simulink model "MKZ_Model"  (R2020a)
settings: Solver=FixedStepAuto  StartTime=0.0  StopTime=RunTime  FixedStep=SampleTime  RelTol=1e-3
PreLoadFcn:
  | load('BrkEngMaps.mat');
values from neighbouring files (symbols this model uses):
  InitVel = VehSpeed.Data(1)    [TestCarModel.m]
  SampleTime = 0.05    [TestCarModel.m]
undefined symbols (not defined in the file or in its folder): BrakeZ, DiscIntNeverNeededParam, EngineZ, XbrkPts, XengPts, YbrkPts, YengPts
libraries: dspstat3 x1
settings Model: Creator=VVK Desktop1  LastModifiedBy=VVK

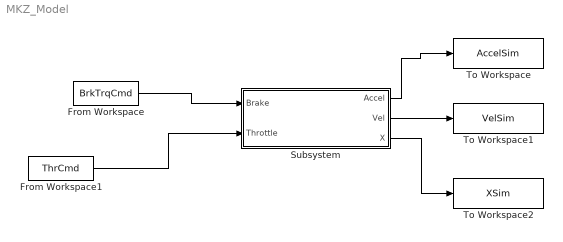
== system MKZ_Model ==
  From Workspace : FromWorkspace  VariableName=BrkTrqCmd  SampleTime=SampleTime
  From Workspace1 : FromWorkspace  VariableName=ThrCmd  SampleTime=SampleTime
  Subsystem : Subsystem
  To Workspace : ToWorkspace  VariableName=AccelSim  SaveFormat=Timeseries  SampleTime=-1
  To Workspace1 : ToWorkspace  VariableName=VelSim  SaveFormat=Timeseries  SampleTime=-1
  To Workspace2 : ToWorkspace  VariableName=XSim  SaveFormat=Timeseries  SampleTime=-1
  wires:
  From Workspace/1 -> Subsystem/1(Brake)
  From Workspace1/1 -> Subsystem/2(Throttle)
  Subsystem/2(Vel) -> To Workspace1/1
  Subsystem/3(X) -> To Workspace2/1
  Subsystem/1(Accel) -> To Workspace/1

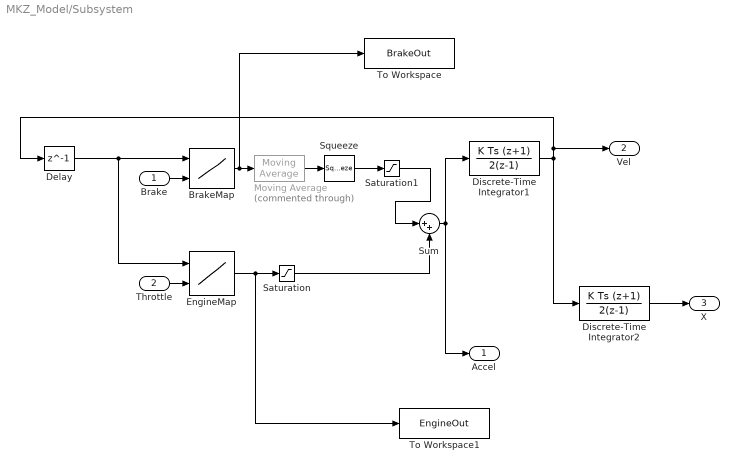
== system MKZ_Model/Subsystem ==
  Brake : Inport
  Throttle : Inport  Port=2
  BrakeMap : Lookup_n-D  BreakpointsForDimension1=XbrkPts  BreakpointsForDimension2=YbrkPts  Table=BrakeZ  InternalRulePriority=Speed  RndMeth=Simplest  InputSameDT=on
  Delay : Delay  DelayLength=1  InitialCondition=InitVel
  Discrete-Time Integrator1 : DiscreteIntegrator  IntegratorMethod=Integration: Trapezoidal  InitialCondition=InitVel  SampleTime=-1  LimitOutput=on  LowerSaturationLimit=0  ICPrevOutput=DiscIntNeverNeededParam  ICPrevScaledInput=DiscIntNeverNeededParam
  Discrete-Time Integrator2 : DiscreteIntegrator  IntegratorMethod=Integration: Trapezoidal  SampleTime=-1  LimitOutput=on  LowerSaturationLimit=0  ICPrevOutput=DiscIntNeverNeededParam  ICPrevScaledInput=DiscIntNeverNeededParam
  EngineMap : Lookup_n-D  BreakpointsForDimension1=XengPts  BreakpointsForDimension2=YengPts  Table=EngineZ  InternalRulePriority=Speed  RndMeth=Simplest  InputSameDT=on
  Moving Average : dspstat3/Moving Average  Commented=through  Method=Sliding window  ForgettingFactorPort=off  SpecifyWindowLength=on  WindowLength=4  ForgettingFactor=0.9  SimulateUsing=Code generation
  Saturation : Saturate  UpperLimit=3.5  LowerLimit=-0.25
  Saturation1 : Saturate  UpperLimit=0  LowerLimit=-3.5
  Squeeze : Squeeze
  Sum : Sum  Inputs=|++
  To Workspace : ToWorkspace  VariableName=BrakeOut  SaveFormat=Timeseries  SampleTime=-1
  To Workspace1 : ToWorkspace  VariableName=EngineOut  SaveFormat=Timeseries  SampleTime=-1
  Accel : Outport
  Vel : Outport  Port=2
  X : Outport  Port=3
  wires:
  Sum/1 -> Accel/1, Discrete-Time Integrator1/1
  Discrete-Time Integrator1/1 -> Discrete-Time Integrator2/1, Delay/1, Vel/1
  Delay/1 -> EngineMap/1, BrakeMap/1
  EngineMap/1 -> To Workspace1/1, Saturation/1
  Brake/1 -> BrakeMap/2
  Discrete-Time Integrator2/1 -> X/1
  Throttle/1 -> EngineMap/2
  Saturation/1 -> Sum/2
  Saturation1/1 -> Sum/1
  BrakeMap/1 -> Moving Average/1, To Workspace/1
  Squeeze/1 -> Saturation1/1
  Moving Average/1 -> Squeeze/1
